simulink model "Project1_s1"  (R2025b)
settings: Solver=ode1  StartTime=0.0  StopTime=25  FixedStep=0.01  RelTol=1e-3
undefined symbols (not defined in the file or in its folder): A, omega0, useSine, w
settings Model: Creator=KI5UXW  LastModifiedBy=KI5UXW

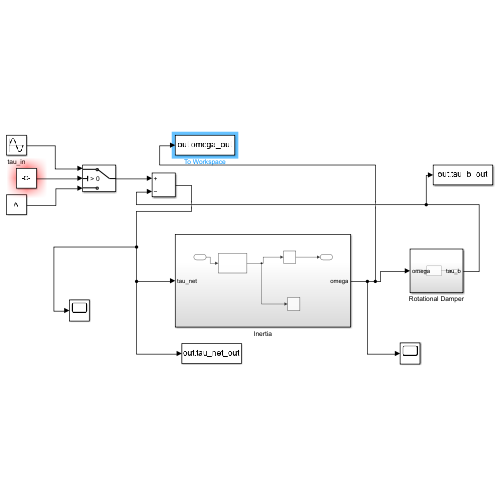
[thumbnail: Simulink's stored preview of the top-level diagram]
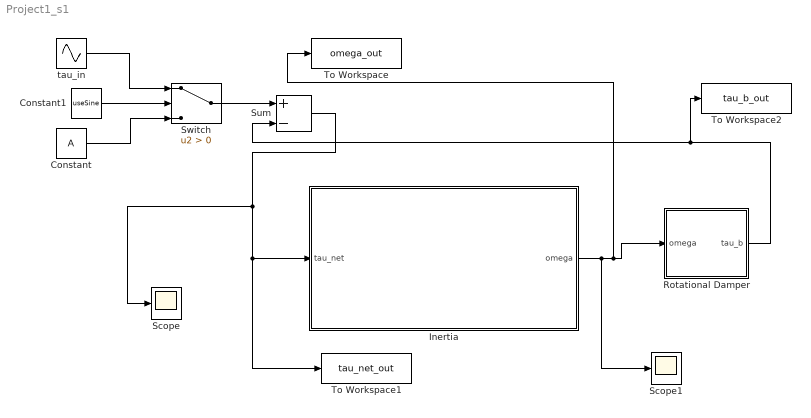
== system Project1_s1 ==
  Constant : Constant  Value=A
  Constant1 : Constant  Value=useSine
  Inertia : Subsystem
  Rotational Damper : Subsystem
  Scope : Scope
      settings: ActiveDisplayYMinimum=-2.1217981751184507E+299  ActiveDisplayYMaximum=2.3125120453084478E+299
  Scope1 : Scope
      settings: ActiveDisplayYMinimum=-1.6261398174868091  ActiveDisplayYMaximum=11.498860182352466  DataLoggingVariableName=ScopeData2
  Sum : Sum  Inputs=+-
  Switch : Switch  Criteria=u2 > Threshold  SaturateOnIntegerOverflow=off  InputSameDT=off
  To Workspace : ToWorkspace  VariableName=omega_out  SaveFormat=Timeseries  SampleTime=-1
  To Workspace1 : ToWorkspace  VariableName=tau_net_out  SaveFormat=Timeseries  SampleTime=-1
  To Workspace2 : ToWorkspace  VariableName=tau_b_out  SaveFormat=Timeseries  SampleTime=-1
  tau_in : Sin  Amplitude=A  Frequency=w  SampleTime=0
  wires:
  Sum/1 -> Scope/1, Inertia/1(tau_net), To Workspace1/1
  Inertia/1(omega) -> Scope1/1, To Workspace/1, Rotational Damper/1(omega)
  Rotational Damper/1(tau_b) -> To Workspace2/1, Sum/2
  Constant/1 -> Switch/3
  tau_in/1 -> Switch/1
  Constant1/1 -> Switch/2
  Switch/1 -> Sum/1

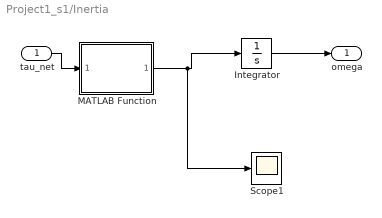
== system Project1_s1/Inertia ==
  tau_net : Inport
  Integrator : Integrator  InitialCondition=omega0
  MATLAB Function : MATLAB Function  TreatAsAtomicUnit=on
  Scope1 : Scope
      settings: ActiveDisplayYMinimum=-1.1147406577554593  ActiveDisplayYMaximum=0.032665919799133816
  omega : Outport
  wires:
  tau_net/1 -> MATLAB Function/1(tau_net)
  MATLAB Function/1(domega) -> Scope1/1, Integrator/1
  Integrator/1 -> omega/1

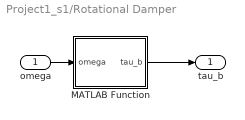
== system Project1_s1/Rotational Damper ==
  omega : Inport
  MATLAB Function : MATLAB Function  TreatAsAtomicUnit=on
  tau_b : Outport
  wires:
  omega/1 -> MATLAB Function/1(omega)
  MATLAB Function/1(tau_b) -> tau_b/1

== matlab function Project1_s1/Inertia/MATLAB Function ==
  data: tau_net input; domega output; J parameter double size=1
function domega = inertia(tau_net, J)

domega = tau_net / J;

== matlab function Project1_s1/Rotational Damper/MATLAB Function ==
  data: omega input; tau_b output; b parameter double size=1
function tau_b = damper(omega, b)

tau_b = b * omega;
